simulink model "Vibration modelling approach2"  (R2021a)
settings: Solver=VariableStepAuto  StartTime=0.0  StopTime=10.0  RelTol=1e-3
settings Model: Creator=mluser  LastModifiedBy=mluser

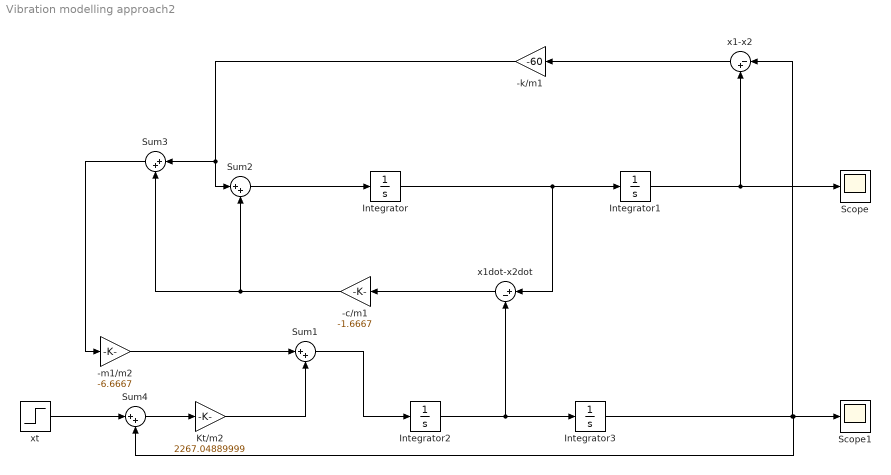
== system Vibration modelling approach2 ==
  -c/m1 : Gain  Gain=-1.6667
  -k/m1 : Gain  Gain=-60
  -m1/m2 : Gain  Gain=-6.6667
  Integrator{,1..3} (4 alike) : Integrator
  Kt/m2 : Gain  Gain=2267.04889999
  Scope : Scope
  Scope1 : Scope
  Sum{1..4} (4 alike) : Sum  Inputs=|++
  x1-x2 : Sum  Inputs=|-+
  x1dot-x2dot : Sum  Inputs=|+-
  xt : Step  SampleTime=0
  wires:
  Integrator2/1 -> x1dot-x2dot/2, Integrator3/1
  Integrator3/1 -> x1-x2/1, Sum4/2, Scope1/1
  Integrator/1 -> x1dot-x2dot/1, Integrator1/1
  Integrator1/1 -> x1-x2/2, Scope/1
  x1dot-x2dot/1 -> -c/m1/1
  x1-x2/1 -> -k/m1/1
  -k/m1/1 -> Sum2/1, Sum3/1
  -c/m1/1 -> Sum2/2, Sum3/2
  Sum2/1 -> Integrator/1
  Sum4/1 -> Kt/m2/1
  xt/1 -> Sum4/1
  Sum3/1 -> -m1/m2/1
  Kt/m2/1 -> Sum1/2
  -m1/m2/1 -> Sum1/1
  Sum1/1 -> Integrator2/1
